simulink model "test_step"  (R2015a)
settings: Solver=ode3  StartTime=0.0  StopTime=SIMEND  FixedStep=ST  RelTol=1e-3
undefined symbols (not defined in the file): den, num
settings Model: Creator=yoshi  LastModifiedBy=yoshi

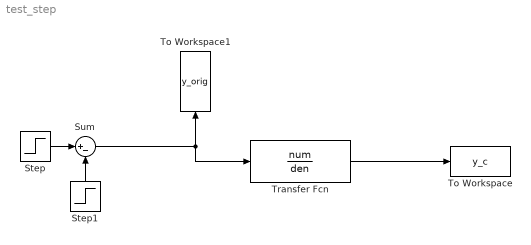
== system test_step ==
  Step : Step  Time=2
  Step1 : Step  Time=4
  Sum : Sum  Inputs=|+-
  To Workspace : ToWorkspace  VariableName=y_c  SaveFormat=Timeseries  SampleTime=-1
  To Workspace1 : ToWorkspace  VariableName=y_orig  SaveFormat=Timeseries  SampleTime=-1
  Transfer Fcn : TransferFcn  Numerator=num  Denominator=den
  wires:
  Sum/1 -> Transfer Fcn/1, To Workspace1/1
  Transfer Fcn/1 -> To Workspace/1
  Step/1 -> Sum/1
  Step1/1 -> Sum/2
  ? -> ?
